simulink library "util_frame_rotation_lib"  (R2015b)
settings: Solver=ode45  SolverMode=SingleTasking  StartTime=0.0  StopTime=10.0  RelTol=1e-3
values from neighbouring files (symbols this model uses):
  D = P*P*P + Q*Q    [mci2lla.m]
undefined symbols (not defined in the file or in its folder): central_body_omega_dot, de_cos_coeff, de_t_poly, e10coeff, e11coeff, e12coeff, e13coeff, e1coeff, e2coeff, e3coeff, e4coeff, e5coeff, e6coeff, e7coeff, e8coeff, e9coeff, earth_moon_rotation_matrix_select, ini_epoch_seconds, ini_hour, ini_minute, ini_moon_rotation_rate, ini_quat_mcmf_to_topo, ini_seconds, ini_tgt_landing_mcmf_pos, omega_moon_iau_coeff, omega_pa_mat_init, ra_sin_coeff, ra_t_poly
undefined symbols (not defined in the file): central_body_flattening, central_body_radius, central_body_rotation_rate
libraries: util_quat_lib x42, util_info_lib x21, util_common_lib x18, util_frame_rotation_lib x14, simulink_extras x9, util_extra_lib x4, simulink x2, util_orbit_dynamics_lib x1
(part 1 of 2)
settings Model: Creator=Administrator  LastModifiedBy=Mark Agbayani
settings DataIOCC: SaveFormat=Array  SignalLoggingSaveFormat=ModelDataLogs
settings OptimizationCC: BlockReduction=off  BooleanDataType=off  ExpressionDepthLimit=2147483647
settings DebuggingCC: SaveWithParameterizedLinksMsg=none  UnderspecifiedInitializationDetection=Classic  MergeDetectMultiDrivingBlocksExec=none  SignalResolutionControl=TryResolveAllWithWarning  FcnCallInpInsideContextMsg=EnableAllAsWarning  StateNameClashWarn=warning  StrictBusMsg=Warning
settings HardwareCC: ProdBitPerPointer=32  ProdLargestAtomicFloat=None  ProdIntDivRoundTo=Undefined  ProdEndianess=Unspecified  ProdWordSize=32  ProdHWDeviceType=32-bit Generic  TargetUnknown=on
settings GRTTargetCC: GeneratePreprocessorConditionals=Disable all
settings ConfigComp: CovModelRefEnable=Off  CovSFcnEnable=off

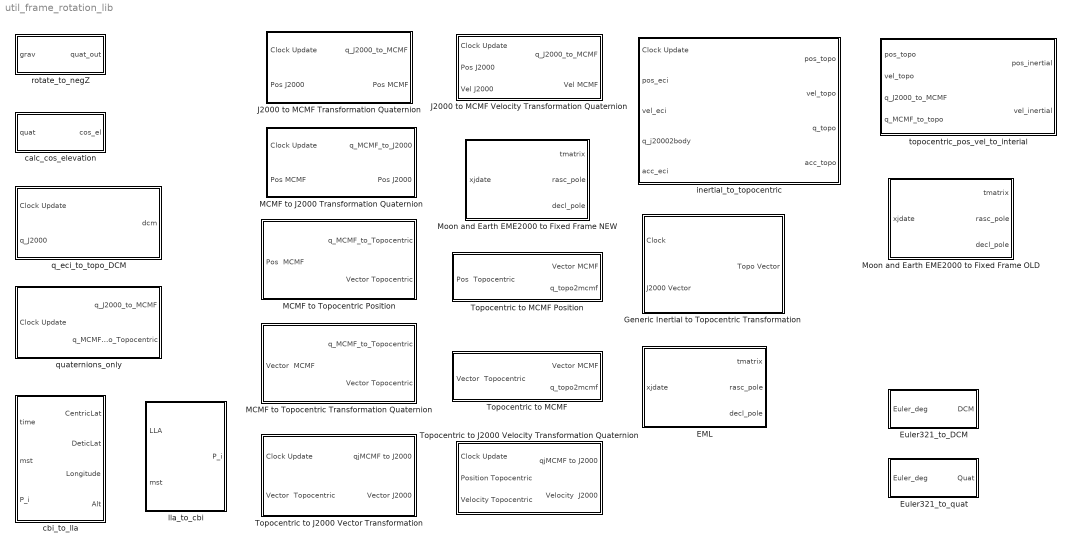
== system util_frame_rotation_lib ==
  EML : Subsystem
      mask Display:
      | color('blue')
      | text(0.05,0.02,'MoonEx',...
      |  	'HorizontalAlignment','Left',...
      | 	'VerticalAlignment','bottom')
  Euler321_to_DCM : Subsystem
  Euler321_to_quat : Subsystem
  Generic Inertial to Topocentric Transformation : Subsystem
  J2000 to MCMF Transformation Quaternion : Subsystem
      mask Display:
      | color('blue')
      | text(0.05,0.02,'MoonEx',...
      |  	'HorizontalAlignment','Left',...
      | 	'VerticalAlignment','bottom')
  J2000 to MCMF Velocity Transformation Quaternion : Subsystem
      mask Display:
      | color('blue')
      | text(0.05,0.02,'MoonEx',...
      |  	'HorizontalAlignment','Left',...
      | 	'VerticalAlignment','bottom')
  MCMF to J2000 Transformation Quaternion : Subsystem
  MCMF to Topocentric Position : Subsystem
      mask Display:
      | color('blue')
      | text(0.05,0.02,'MoonEx',...
      |  	'HorizontalAlignment','Left',...
      | 	'VerticalAlignment','bottom')
  MCMF to Topocentric Transformation Quaternion : Subsystem
      mask Display:
      | color('blue')
      | text(0.05,0.02,'MoonEx',...
      |  	'HorizontalAlignment','Left',...
      | 	'VerticalAlignment','bottom')
  Moon and Earth EME2000 to Fixed Frame NEW : Subsystem
      mask Display:
      | color('blue')
      | text(0.05,0.02,'MoonEx',...
      |  	'HorizontalAlignment','Left',...
      | 	'VerticalAlignment','bottom')
  Moon and Earth EME2000 to Fixed Frame OLD : Subsystem
      mask Display:
      | color('blue')
      | text(0.05,0.02,'MoonEx',...
      |  	'HorizontalAlignment','Left',...
      | 	'VerticalAlignment','bottom')
  "Topocentric to J2000 Vector Transformation " : Subsystem
      mask Display:
      | color('blue')
      | text(0.05,0.02,'MoonEx',...
      |  	'HorizontalAlignment','Left',...
      | 	'VerticalAlignment','bottom')
  Topocentric to J2000 Velocity Transformation Quaternion : Subsystem  TreatAsAtomicUnit=on
      mask Display:
      | color('blue')
      | text(0.05,0.02,'MoonEx',...
      |  	'HorizontalAlignment','Left',...
      | 	'VerticalAlignment','bottom')
  Topocentric to MCMF : Subsystem
      mask Display:
      | color('blue')
      | text(0.05,0.02,'MoonEx',...
      |  	'HorizontalAlignment','Left',...
      | 	'VerticalAlignment','bottom')
  Topocentric to MCMF Position : Subsystem
      mask Display:
      | color('blue')
      | text(0.05,0.02,'MoonEx',...
      |  	'HorizontalAlignment','Left',...
      | 	'VerticalAlignment','bottom')
  calc_cos_elevation : Subsystem
  cbi_to_lla : Subsystem  mask{a=central_body_radius, b=central_body_radius*(1-central_body_flattening), omega=central_body_rotation_rate(3)}
      mask prompts: a "Central Body Semi-major Axis (Equatorial Radius), a [m]"; b "Central Body Semi-minor Axis (Polar Radius), b [m]"; omega "Central Body Rotation Rate, omega [rad/s]"
      mask help:
      | FUNCTION cbi_to_lla
      |   Compute Detic Latitude, Centric Latitude, Longitude, and Detic Altitude
      |   from Central Body Inertial Coordinates
      |
      |   [latD, latC, lon, alt] = cbi_to_lla( P_i, t, mst)
      |
      | INPUTS
      |   P_i      [1x3]   [m]         Position in Central Body Inertial Frame
      |   mst      [1x1]   [degrees]   Mean Sidereal Time of Epoch
      |   time     [1x1]   [sec]       Time Since Epoch
      |
      | OUTPUTS
      |   latC     [1x1]   [deg]       Centric Latitude
      |   latD     [1x1]   [deg]       Detic Latitude
      |   lon      [1x1]   [deg]       Longitude
      |   alt      [1x1]   [m]         Detic Altitude
      mask init:
      | flatten = 1 - b/a;
      mask Display:
      | color('blue')
      | text(0.05,0.02,'MoonEx',...
      |  	'HorizontalAlignment','Left',...
      | 	'VerticalAlignment','bottom')
  inertial_to_topocentric : Subsystem
      mask Display:
      | color('blue')
      | text(0.05,0.02,'MoonEx',...
      |  	'HorizontalAlignment','Left',...
      | 	'VerticalAlignment','bottom')
  lla_to_cbi : Subsystem  mask{a=central_body_radius, b=central_body_radius*(1-central_body_flattening)}
      mask prompts: a "Central Body Semi-major Axis (Equatorial Radius), a [m]"; b "Central Body Semi-minor Axis (Polar Radius), b [m]"
      mask help:
      | FUNCTION lla_to_cbi
      |   Converts Detic Latitude, Longitude, and Altitude
      |   to Central Body Inertial Coordinates.
      |
      |   P_i = lla_to_cbi( LLA, mst)
      |
      | INPUTS
      |   LLA      [1x3]   [deg deg m]    Detic Lattitude, Longitude, Altitude
      |   mst      [1x1]   [degrees]      Mean Sidereal Time of Epoch
      |
      | OUTPUTS
      |   P_i      [1x3]   [m]            Position in Central Body Inertial Frame
      mask init:
      | flatten = 1 - b/a;
      mask Display:
      | color('blue')
      | text(0.05,0.02,'MoonEx',...
      |  	'HorizontalAlignment','Left',...
      | 	'VerticalAlignment','bottom')
  q_eci_to_topo_DCM : Subsystem
      mask Display:
      | color('blue')
      | text(0.05,0.02,'MoonEx',...
      |  	'HorizontalAlignment','Left',...
      | 	'VerticalAlignment','bottom')
  quaternions_only : Subsystem
      mask Display:
      | color('blue')
      | text(0.05,0.02,'MoonEx',...
      |  	'HorizontalAlignment','Left',...
      | 	'VerticalAlignment','bottom')
  rotate_to_negZ : Subsystem
  topocentric_pos_vel_to_interial : Subsystem
      mask Display:
      | color('blue')
      | text(0.05,0.02,'MoonEx',...
      |  	'HorizontalAlignment','Left',...
      | 	'VerticalAlignment','bottom')

== system util_frame_rotation_lib/EML ==
  xjdate : Inport
  EME2000 (J2000) to Moon Centered Moon Fixed (MCMF) : MATLAB Function  TreatAsAtomicUnit=on
  Library Information : util_info_lib/Library Information  owner='NONE'
  Moon Rotation Rate vector : Constant  Value=ini_moon_rotation_rate
  tmatrix : Outport
  rasc_pole : Outport  Port=2
  decl_pole : Outport  Port=3
  wires:
  EME2000 (J2000) to Moon Centered Moon Fixed (MCMF)/1(tmatrix) -> tmatrix/1
  EME2000 (J2000) to Moon Centered Moon Fixed (MCMF)/2(rasc_pole) -> rasc_pole/1
  EME2000 (J2000) to Moon Centered Moon Fixed (MCMF)/3(decl_pole) -> decl_pole/1
  xjdate/1 -> EME2000 (J2000) to Moon Centered Moon Fixed (MCMF)/1(xjdate)
  Moon Rotation Rate vector/1 -> EME2000 (J2000) to Moon Centered Moon Fixed (MCMF)/2(moonrotationrate)

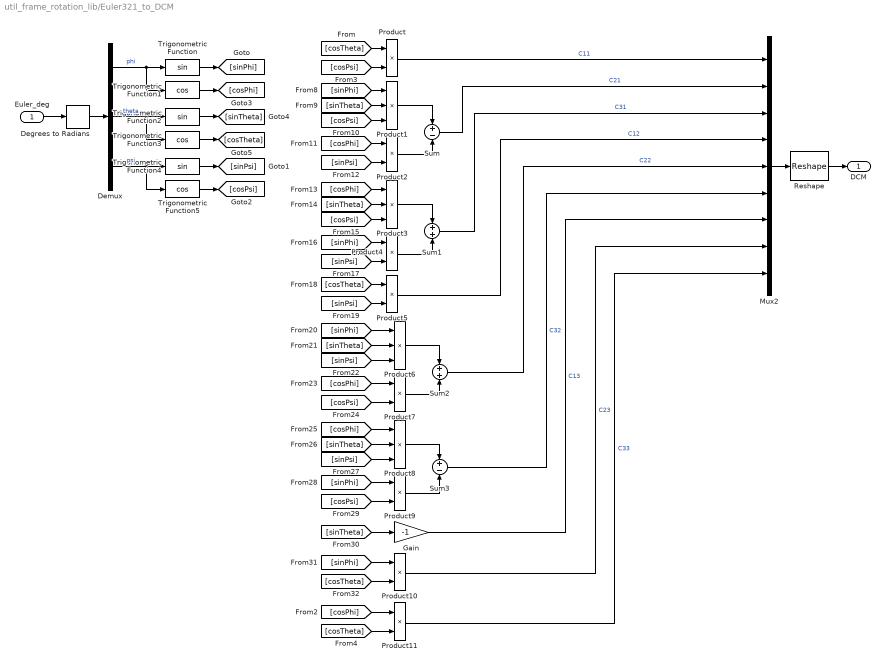
== system util_frame_rotation_lib/Euler321_to_DCM ==
  Euler_deg : Inport
  Degrees to Radians : simulink_extras/Transformations/Degrees to Radians
  Demux : Demux  Outputs=3
  Gain : Gain  Gain=-1
  Mux2 : Mux  Inputs=9
  Product{,2,4..5,7,9..11} (8 alike) : Product  RndMeth=Zero
  Product{1,3,6,8} (4 alike) : Product  Inputs=3  RndMeth=Zero
  Reshape : Reshape  OutputDimensionality=Customize  OutputDimensions=[3,3]
  Sum : Sum  Inputs=+|-
  Sum1 : Sum  Inputs=+|+
  Sum2 : Sum  Inputs=+|+
  Sum3 : Sum  Inputs=+|-
  Trigonometric Function : Trigonometry
  Trigonometric Function1 : Trigonometry  Operator=cos
  Trigonometric Function2 : Trigonometry
  Trigonometric Function3 : Trigonometry  Operator=cos
  Trigonometric Function4 : Trigonometry
  Trigonometric Function5 : Trigonometry  Operator=cos
  DCM : Outport
  wires:
  Degrees to Radians/1 -> Demux/1
  Demux/1 -> Trigonometric Function/1, Trigonometric Function1/1  "phi"
  Demux/2 -> Trigonometric Function3/1, Trigonometric Function2/1  "theta"
  Demux/3 -> Trigonometric Function4/1, Trigonometric Function5/1  "psi"
  Trigonometric Function/1 -> [sinPhi]
  Trigonometric Function1/1 -> [cosPhi]
  Trigonometric Function2/1 -> [sinTheta]
  Trigonometric Function3/1 -> [cosTheta]
  Trigonometric Function4/1 -> [sinPsi]
  Trigonometric Function5/1 -> [cosPsi]
  [cosTheta] -> Product/1
  [cosPsi] -> Product/2
  Product/1 -> Mux2/1  "C11"
  Product1/1 -> Sum/1
  Product2/1 -> Sum/2
  [sinPhi] -> Product1/1
  [sinTheta] -> Product1/2
  [cosPsi] -> Product1/3
  [cosPhi] -> Product2/1
  [sinPsi] -> Product2/2
  Sum/1 -> Mux2/2  "C21"
  Product3/1 -> Sum1/1
  Product4/1 -> Sum1/2
  Sum1/1 -> Mux2/3  "C31"
  [cosPhi] -> Product3/1
  [sinTheta] -> Product3/2
  [cosPsi] -> Product3/3
  [sinPhi] -> Product4/1
  [sinPsi] -> Product4/2
  [cosTheta] -> Product5/1
  [sinPsi] -> Product5/2
  Product5/1 -> Mux2/4  "C12"
  Product6/1 -> Sum2/1
  Product7/1 -> Sum2/2
  [sinPhi] -> Product6/1
  [sinTheta] -> Product6/2
  [sinPsi] -> Product6/3
  [cosPhi] -> Product7/1
  [cosPsi] -> Product7/2
  Sum2/1 -> Mux2/5  "C22"
  Product8/1 -> Sum3/1
  Product9/1 -> Sum3/2
  [cosPhi] -> Product8/1
  [sinTheta] -> Product8/2
  [sinPsi] -> Product8/3
  [sinPhi] -> Product9/1
  [cosPsi] -> Product9/2
  Sum3/1 -> Mux2/6  "C32"
  Gain/1 -> Mux2/7  "C13"
  [sinTheta] -> Gain/1
  [sinPhi] -> Product10/1
  [cosTheta] -> Product10/2
  Product10/1 -> Mux2/8  "C23"
  [cosPhi] -> Product11/1
  [cosTheta] -> Product11/2
  Product11/1 -> Mux2/9  "C33"
  Euler_deg/1 -> Degrees to Radians/1
  Mux2/1 -> Reshape/1
  Reshape/1 -> DCM/1

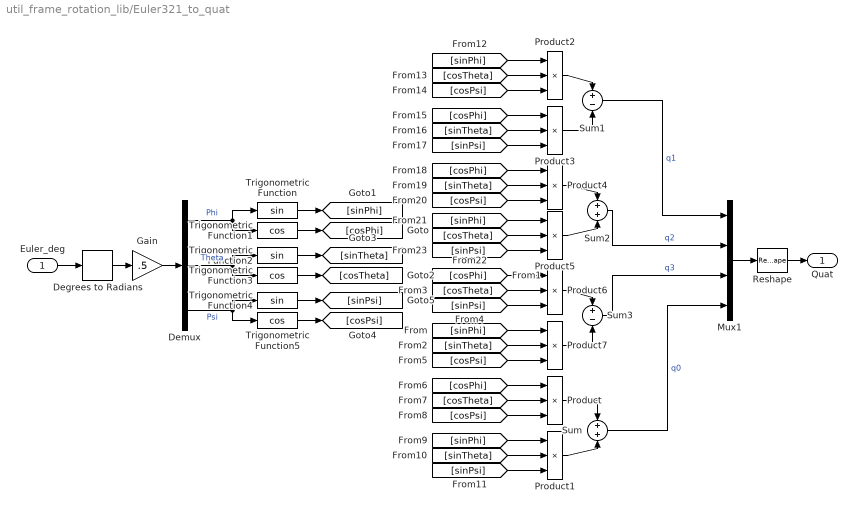
== system util_frame_rotation_lib/Euler321_to_quat ==
  Euler_deg : Inport
  Degrees to Radians : simulink_extras/Transformations/Degrees to Radians
  Demux : Demux  Outputs=3
  Gain : Gain  Gain=.5
  Mux1 : Mux
  Product{,1..7} (8 alike) : Product  Inputs=3  RndMeth=Zero
  Reshape : Reshape
  Sum : Sum  Inputs=+|+
  Sum1 : Sum  Inputs=+|-
  Sum2 : Sum  Inputs=+|+
  Sum3 : Sum  Inputs=+|-
  Trigonometric Function : Trigonometry
  Trigonometric Function1 : Trigonometry  Operator=cos
  Trigonometric Function2 : Trigonometry
  Trigonometric Function3 : Trigonometry  Operator=cos
  Trigonometric Function4 : Trigonometry
  Trigonometric Function5 : Trigonometry  Operator=cos
  Quat : Outport
  wires:
  Reshape/1 -> Quat/1
  Mux1/1 -> Reshape/1
  Euler_deg/1 -> Degrees to Radians/1
  [cosPsi] -> Product7/3
  [sinTheta] -> Product7/2
  [sinPhi] -> Product7/1
  [sinPsi] -> Product6/3
  [cosTheta] -> Product6/2
  [cosPhi] -> Product6/1
  Product6/1 -> Sum3/1
  Product7/1 -> Sum3/2
  Product5/1 -> Sum2/2
  [sinPsi] -> Product5/3
  [cosTheta] -> Product5/2
  [sinPhi] -> Product5/1
  Product4/1 -> Sum2/1
  [cosPsi] -> Product4/3
  [sinTheta] -> Product4/2
  [cosPhi] -> Product4/1
  Product3/1 -> Sum1/2
  [sinPsi] -> Product3/3
  [sinTheta] -> Product3/2
  [cosPhi] -> Product3/1
  Product2/1 -> Sum1/1
  [cosPsi] -> Product2/3
  [cosTheta] -> Product2/2
  [sinPhi] -> Product2/1
  [sinPsi] -> Product1/3
  [sinTheta] -> Product1/2
  [sinPhi] -> Product1/1
  Product1/1 -> Sum/2
  Product/1 -> Sum/1
  [cosPsi] -> Product/3
  [cosTheta] -> Product/2
  [cosPhi] -> Product/1
  Trigonometric Function5/1 -> [cosPsi]
  Trigonometric Function4/1 -> [sinPsi]
  Trigonometric Function3/1 -> [cosTheta]
  Trigonometric Function2/1 -> [sinTheta]
  Trigonometric Function1/1 -> [cosPhi]
  Trigonometric Function/1 -> [sinPhi]
  Demux/3 -> Trigonometric Function5/1, Trigonometric Function4/1  "Psi"
  Demux/2 -> Trigonometric Function3/1, Trigonometric Function2/1  "Theta"
  Demux/1 -> Trigonometric Function1/1, Trigonometric Function/1  "Phi"
  Gain/1 -> Demux/1
  Sum1/1 -> Mux1/1  "q1"
  Sum2/1 -> Mux1/2  "q2"
  Sum3/1 -> Mux1/3  "q3"
  Sum/1 -> Mux1/4  "q0"
  Degrees to Radians/1 -> Gain/1

== system util_frame_rotation_lib/Generic Inertial to Topocentric Transformation ==
  Clock : Inport
  J2000 Vector : Inport  Port=2
  J2000 to MCMF Transformation Quaternion1 : util_frame_rotation_lib/J2000 to MCMF  Transformation Quaternion  SystemSampleTime=-1
  Library Information : util_info_lib/Library Information  owner='NONE'
  MCMF to Topocentric Transformation Quaternion : util_frame_rotation_lib/MCMF to Topocentric  Transformation Quaternion  SystemSampleTime=-1
  Terminator : Terminator
  Terminator1 : Terminator
  Topo Vector : Outport
  wires:
  J2000 to MCMF Transformation Quaternion1/2 -> MCMF to Topocentric Transformation Quaternion/1
  J2000 to MCMF Transformation Quaternion1/1 -> Terminator/1
  J2000 Vector/1 -> J2000 to MCMF Transformation Quaternion1/2
  MCMF to Topocentric Transformation Quaternion/2 -> Topo Vector/1
  Clock/1 -> J2000 to MCMF Transformation Quaternion1/1
  MCMF to Topocentric Transformation Quaternion/1 -> Terminator1/1

== system util_frame_rotation_lib/J2000 to MCMF Transformation Quaternion ==
  Clock Update : Inport
  Pos J2000 : Inport  Port=2
  Add : Sum
  Divide : Product  Inputs=*/
  Library Information : util_info_lib/Library Information  owner='NONE'
  Moon and Earth EME2000 to Fixed Frame NEW : util_frame_rotation_lib/Moon and Earth  EME2000 to Fixed Frame NEW  SystemSampleTime=-1
  "Number of Days From Start of Julian Date to Jan 1, 2000 12:00:00" : Constant  Value=2451545
  Number of Seconds Per Day : Constant  Description=|  Value=86400
      | Number of Seconds                   
      | July 4, 2014 22:40:00 UTC           
      | Calculate on Web Site:              
      | www.mbari.org/staff/rich/utccalc.htm
  Terminator1 : Terminator
  Terminator5 : Terminator
  quaternion_frame_transformation : util_quat_lib/quaternion_frame_transformation  SystemSampleTime=-1
  rotm_to_quaternion EME2000 to MCMF : util_extra_lib/rotm_to_quaternion
  q_J2000_to_MCMF : Outport
  Pos MCMF : Outport  Port=2
  wires:
  Moon and Earth EME2000 to Fixed Frame NEW/1 -> rotm_to_quaternion EME2000 to MCMF/1
  Number of Seconds Per Day/1 -> Divide/2
  rotm_to_quaternion EME2000 to MCMF/1 -> quaternion_frame_transformation/2, q_J2000_to_MCMF/1
  Clock Update/1 -> Divide/1  "Seconds Since Jan 1, 2000  12:00:00"
  quaternion_frame_transformation/1 -> Pos MCMF/1
  "Number of Days From Start of Julian Date to Jan 1, 2000 12:00:00"/1 -> Add/2
  Moon and Earth EME2000 to Fixed Frame NEW/2 -> Terminator5/1
  Moon and Earth EME2000 to Fixed Frame NEW/3 -> Terminator1/1
  Add/1 -> Moon and Earth EME2000 to Fixed Frame NEW/1
  Divide/1 -> Add/1
  Pos J2000/1 -> quaternion_frame_transformation/1

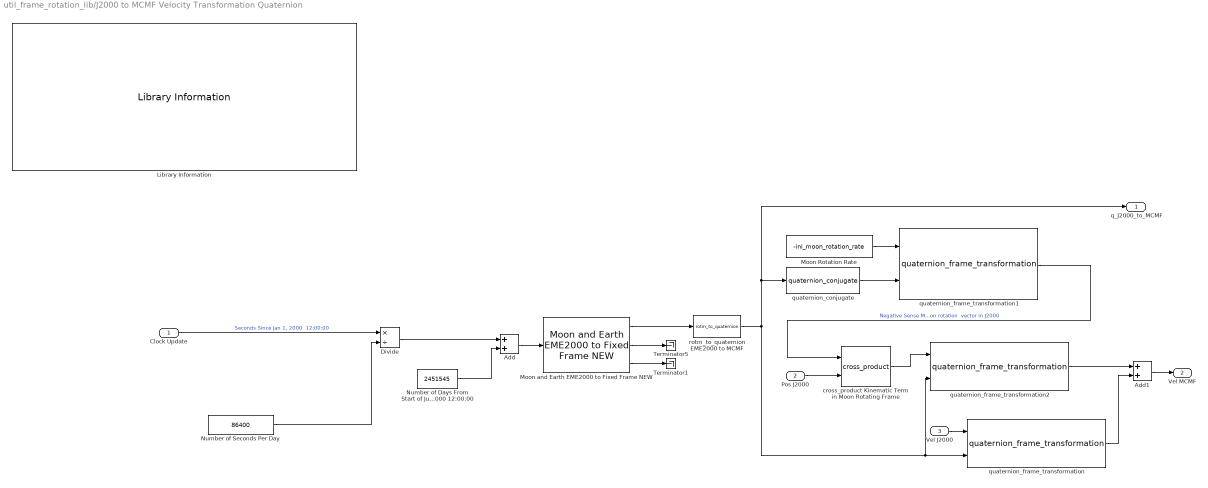
== system util_frame_rotation_lib/J2000 to MCMF Velocity Transformation Quaternion ==
  Clock Update : Inport
  Pos J2000 : Inport  Port=2
  Vel J2000 : Inport  Port=3
  Add : Sum
  Add1 : Sum
  Divide : Product  Inputs=*/
  Library Information : util_info_lib/Library Information  owner='NONE'
  Moon Rotation Rate : Constant  Value=-ini_moon_rotation_rate
  Moon and Earth EME2000 to Fixed Frame NEW : util_frame_rotation_lib/Moon and Earth  EME2000 to Fixed Frame NEW  SystemSampleTime=-1
  "Number of Days From Start of Julian Date to Jan 1, 2000 12:00:00" : Constant  Value=2451545
  Number of Seconds Per Day : Constant  Description=|  Value=86400
      | Number of Seconds                   
      | July 4, 2014 22:40:00 UTC           
      | Calculate on Web Site:              
      | www.mbari.org/staff/rich/utccalc.htm
  Terminator1 : Terminator
  Terminator5 : Terminator
  cross_product Kinematic Term in Moon Rotating Frame : util_common_lib/cross_product  SystemSampleTime=-1
  quaternion_conjugate : util_quat_lib/quaternion_conjugate  SystemSampleTime=-1
  quaternion_frame_transformation : util_quat_lib/quaternion_frame_transformation  SystemSampleTime=-1
  quaternion_frame_transformation1 : util_quat_lib/quaternion_frame_transformation  SystemSampleTime=-1
  quaternion_frame_transformation2 : util_quat_lib/quaternion_frame_transformation  SystemSampleTime=-1
  rotm_to_quaternion EME2000 to MCMF : util_extra_lib/rotm_to_quaternion
  q_J2000_to_MCMF : Outport
  Vel MCMF : Outport  Port=2
  wires:
  Vel J2000/1 -> quaternion_frame_transformation/1
  Divide/1 -> Add/1
  Add/1 -> Moon and Earth EME2000 to Fixed Frame NEW/1
  Moon and Earth EME2000 to Fixed Frame NEW/3 -> Terminator1/1
  Moon and Earth EME2000 to Fixed Frame NEW/2 -> Terminator5/1
  "Number of Days From Start of Julian Date to Jan 1, 2000 12:00:00"/1 -> Add/2
  Clock Update/1 -> Divide/1  "Seconds Since Jan 1, 2000  12:00:00"
  rotm_to_quaternion EME2000 to MCMF/1 -> quaternion_frame_transformation2/2, quaternion_frame_transformation/2, q_J2000_to_MCMF/1, quaternion_conjugate/1
  Number of Seconds Per Day/1 -> Divide/2
  Moon and Earth EME2000 to Fixed Frame NEW/1 -> rotm_to_quaternion EME2000 to MCMF/1
  Moon Rotation Rate/1 -> quaternion_frame_transformation1/1
  quaternion_conjugate/1 -> quaternion_frame_transformation1/2
  quaternion_frame_transformation1/1 -> cross_product Kinematic Term in Moon Rotating Frame/1  "Negative Sense Moon rotation  vector in J2000"
  Add1/1 -> Vel MCMF/1
  quaternion_frame_transformation/1 -> Add1/2
  Pos J2000/1 -> cross_product Kinematic Term in Moon Rotating Frame/2
  quaternion_frame_transformation2/1 -> Add1/1
  cross_product Kinematic Term in Moon Rotating Frame/1 -> quaternion_frame_transformation2/1

== system util_frame_rotation_lib/MCMF to J2000 Transformation Quaternion ==
  note: Calculate on Web Site:
      | www.mbari.org/staff/rich/utccalc.htm
  Clock Update : Inport
  Pos MCMF : Inport  Port=2
  Add : Sum
  Divide : Product  Inputs=*/
  Library Information : util_info_lib/Library Information  owner='NONE'
  Moon and Earth EME2000 to Fixed Frame NEW : util_frame_rotation_lib/Moon and Earth  EME2000 to Fixed Frame NEW  SystemSampleTime=-1
  "Number of Days From Start of Julian Date to Jan 1, 2000 12:00:00" : Constant  Value=2451545
  Number of Seconds Per Day : Constant  Description=|  Value=86400
      | Number of Seconds                   
      | July 4, 2014 22:40:00 UTC           
      | Calculate on Web Site:              
      | www.mbari.org/staff/rich/utccalc.htm
  Terminator1 : Terminator
  Terminator5 : Terminator
  quaternion_conjugate : util_quat_lib/quaternion_conjugate  SystemSampleTime=-1
  quaternion_frame_transformation : util_quat_lib/quaternion_frame_transformation  SystemSampleTime=-1
  rotm_to_quaternion EME2000 to MCMF : util_extra_lib/rotm_to_quaternion
  q_MCMF_to_J2000 : Outport
  Pos J2000 : Outport  Port=2
  wires:
  Pos MCMF/1 -> quaternion_frame_transformation/1
  Divide/1 -> Add/1
  Add/1 -> Moon and Earth EME2000 to Fixed Frame NEW/1
  Moon and Earth EME2000 to Fixed Frame NEW/3 -> Terminator1/1
  Moon and Earth EME2000 to Fixed Frame NEW/2 -> Terminator5/1
  "Number of Days From Start of Julian Date to Jan 1, 2000 12:00:00"/1 -> Add/2
  quaternion_frame_transformation/1 -> Pos J2000/1
  Clock Update/1 -> Divide/1  "Seconds Since Jan 1, 2000  12:00:00"
  rotm_to_quaternion EME2000 to MCMF/1 -> quaternion_conjugate/1
  Number of Seconds Per Day/1 -> Divide/2
  Moon and Earth EME2000 to Fixed Frame NEW/1 -> rotm_to_quaternion EME2000 to MCMF/1
  quaternion_conjugate/1 -> quaternion_frame_transformation/2, q_MCMF_to_J2000/1

== system util_frame_rotation_lib/MCMF to Topocentric Position ==
  Pos  MCMF : Inport
  Constant10 : Constant  Value=ini_tgt_landing_mcmf_pos
  Library Information : util_info_lib/Library Information  owner='NONE'
  Moon Rotation Rate in MCMF : Constant  Value=ini_quat_mcmf_to_topo
  Subtract1 : Sum  Inputs=-+
  quaternion_frame_transformation1 : util_quat_lib/quaternion_frame_transformation  SystemSampleTime=-1
  q_MCMF_to_Topocentric : Outport
  Vector Topocentric : Outport  Port=2
  wires:
  Moon Rotation Rate in MCMF/1 -> quaternion_frame_transformation1/2, q_MCMF_to_Topocentric/1
  quaternion_frame_transformation1/1 -> Vector Topocentric/1
  Constant10/1 -> Subtract1/1
  Pos  MCMF/1 -> Subtract1/2
  Subtract1/1 -> quaternion_frame_transformation1/1

== system util_frame_rotation_lib/MCMF to Topocentric Transformation Quaternion ==
  Vector  MCMF : Inport
  Library Information : util_info_lib/Library Information  owner='NONE'
  Moon Rotation Rate in MCMF : Constant  Value=ini_quat_mcmf_to_topo
  quaternion_frame_transformation1 : util_quat_lib/quaternion_frame_transformation  SystemSampleTime=-1
  q_MCMF_to_Topocentric : Outport
  Vector Topocentric : Outport  Port=2
  wires:
  Moon Rotation Rate in MCMF/1 -> quaternion_frame_transformation1/2, q_MCMF_to_Topocentric/1
  quaternion_frame_transformation1/1 -> Vector Topocentric/1
  Vector  MCMF/1 -> quaternion_frame_transformation1/1

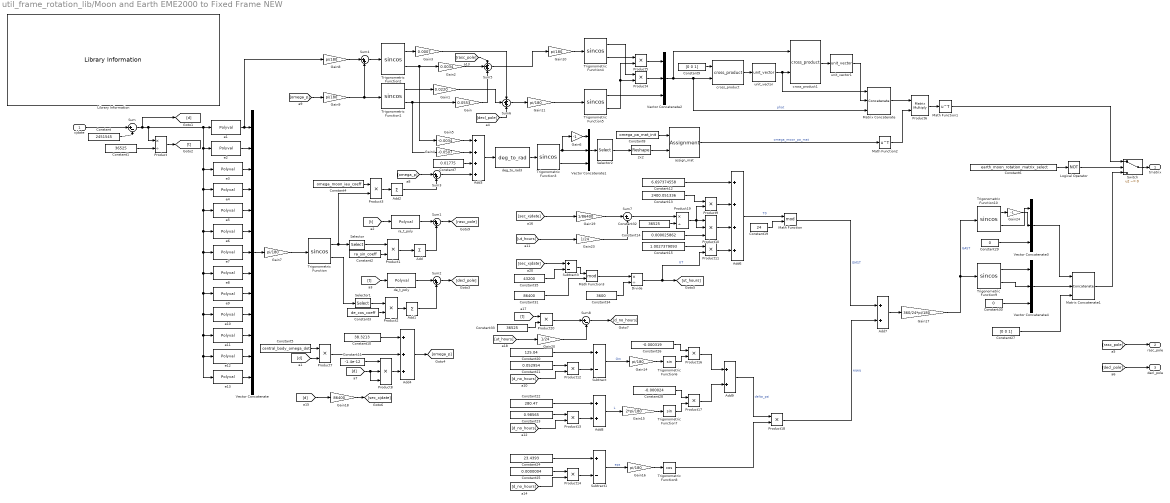
== system util_frame_rotation_lib/Moon and Earth EME2000 to Fixed Frame NEW ==
  xjdate : Inport
  2x2 : Reshape  OutputDimensionality=Customize  OutputDimensions=[2,2]
  Add : Sum  Inputs=+
  Add1 : Sum  Inputs=+
  Add2 : Sum  Inputs=+
  Add3 : Sum  Inputs=4
  Add4 : Sum  Inputs=3
  Add6 : Sum  Inputs=4
  Add7 : Sum  Inputs=2
  Add8 : Sum  Inputs=2
  Add9 : Sum  Inputs=2
  Constant : Constant  Value=2451545
  Constant1 : Constant  Value=36525
  Constant10 : Constant  Value=38.3213
  Constant11 : Constant  Value=-1.4e-12
  Constant12 : Constant  Value=6.697374558
  Constant13 : Constant  Value=2400.051336
  Constant14 : Constant  Value=0.000025862
  Constant15 : Constant  Value=1.0027379093
  Constant19 : Constant  Value=24
  Constant2 : Constant  Value=ra_sin_coeff
  Constant20 : Constant  Value=125.04
  Constant21 : Constant  Value=0.052954
  Constant22 : Constant  Value=280.47
  Constant23 : Constant  Value=0.98565
  Constant24 : Constant  Value=23.4393
  Constant25 : Constant  Value=0.0000004
  Constant26 : Constant  Value=-0.000319
  Constant27 : Constant  Value=[0 0 1]
  Constant28 : Constant  Value=-0.000024
  Constant29 : Constant  Value=0
  Constant3 : Constant  Value=de_cos_coeff
  Constant30 : Constant  Value=0
  Constant31 : Constant  Value=86400
  Constant32 : Constant  Value=36525
  Constant33 : Constant  Value=36525
  Constant34 : Constant  Value=3600
  Constant35 : Constant  Value=43200
  Constant4 : Constant  Value=omega_moon_iau_coeff
  Constant5 : Constant  Value=central_body_omega_dot
  Constant6 : Constant  Value=earth_moon_rotation_matrix_select
  Constant7 : Constant  Value=0.01775
  Constant8 : Constant  Value=omega_pa_mat_init
  Constant9 : Constant  Value=[0 0 1]
  Divide : Product  Inputs=*/
  Gain : Gain  Gain=0.0553
  Gain1 : Gain  Gain=0.0220
  Gain{7..11,14,16} (7 alike) : Gain  Gain=pi/180
  Gain15 : Gain  Gain=2*pi/180
  Gain17 : Gain  Gain=360/24*pi/180
  Gain18 : Gain  Gain=86400
  Gain19 : Gain  Gain=1/86400
  Gain2 : Gain  Gain=0.0034
  Gain20 : Gain  Gain=1/24
  Gain23 : Gain  Gain=1/24
  Gain24 : Gain  Gain=-1
  Gain3 : Gain  Gain=0.0007
  Gain4 : Gain  Gain=-0.0507
  Gain5 : Gain  Gain=-0.0034
  Gain6 : Gain  Gain=-1
  Library Information : util_info_lib/Library Information  owner='escrane'
  Logical Operator : Logic  Operator=NOT  AllPortsSameDT=off  OutDataTypeStr=boolean
  Math Function : Math  Operator=mod  SaturateOnIntegerOverflow=on
  Math Function1 : Math  Operator=transpose  SaturateOnIntegerOverflow=on
  Math Function2 : Math  Operator=transpose  SaturateOnIntegerOverflow=on
  Math Function3 : Math  Operator=mod  SaturateOnIntegerOverflow=on
  Matrix Concatenate : Concatenate  NumInputs=3  Mode=Multidimensional array  ConcatenateDimension=2
  Matrix Concatenate1 : Concatenate  NumInputs=3  Mode=Multidimensional array  ConcatenateDimension=2
  Product : Product  Inputs=*/
  Product{1..5,7,9,11..14,16..18,20} (15 alike) : Product
  Product10 : Product  Inputs=3
  Product19 : Product  Inputs=*/
  Product6 : Product  Multiplication=Matrix(*)
  Product8 : Product  Inputs=3
  Selector : Selector  InputPortWidth=13  IndexOptions=Index vector (dialog)  Indices=[1 2 3 4 6 10 13]  OutputSizes=1
  Selector1 : Selector  InputPortWidth=13  IndexOptions=Index vector (dialog)  Indices=[1 2 3 4 6 7 10 13]  OutputSizes=1
  Selector2 : Selector  InputPortWidth=3  IndexOptions=Index vector (dialog)  Indices=[3 1 2 3]  OutputSizes=1
  Subtract : Sum  Inputs=+-
  Subtract1 : Sum  Inputs=+-
  Subtract3 : Sum  Inputs=+-
  Sum : Sum  Inputs=|+-
  Sum{1..4} (4 alike) : Sum  Inputs=|++
  Sum5 : Sum  Inputs=+++
  Sum6 : Sum  Inputs=+++
  Sum7 : Sum  Inputs=|+-
  Sum8 : Sum  Inputs=|+-
  Switch : Switch  Criteria=u2 ~= 0
  Trigonometric Function{,1..5,9..10} (8 alike) : Trigonometry  Operator=sincos
  Trigonometric Function6 : Trigonometry
  Trigonometric Function7 : Trigonometry
  Trigonometric Function8 : Trigonometry  Operator=cos
  Vector Concatenate : Concatenate  NumInputs=13
  Vector Concatenate{1..4} (4 alike) : Concatenate  NumInputs=3
  assign_mat : Assignment  NumberOfDimensions=2  IndexOptions=Index vector (dialog),Index vector (dialog)  Indices=[1 2],[1 2]  OutputSizes=1,1
  cross_product : util_common_lib/cross_product  SystemSampleTime=-1
  cross_product1 : util_common_lib/cross_product  SystemSampleTime=-1
  de_t_poly : Polyval  Coefs=de_t_poly
  deg_to_rad3 : util_common_lib/deg_to_rad  SystemSampleTime=-1
  e1 : Polyval  Coefs=e1coeff
  e10 : Polyval  Coefs=e10coeff
  e11 : Polyval  Coefs=e11coeff
  e12 : Polyval  Coefs=e12coeff
  e13 : Polyval  Coefs=e13coeff
  e2 : Polyval  Coefs=e2coeff
  e3 : Polyval  Coefs=e3coeff
  e4 : Polyval  Coefs=e4coeff
  e5 : Polyval  Coefs=e5coeff
  e6 : Polyval  Coefs=e6coeff
  e7 : Polyval  Coefs=e7coeff
  e8 : Polyval  Coefs=e8coeff
  e9 : Polyval  Coefs=e9coeff
  ra_t_poly : Polyval  Coefs=ra_t_poly
  unit_vector : util_common_lib/unit_vector  SystemSampleTime=-1
  unit_vector1 : util_common_lib/unit_vector  SystemSampleTime=-1
  tmatrix : Outport
  rasc_pole : Outport  Port=2
  decl_pole : Outport  Port=3
  wires:
  [decl_pole] -> decl_pole/1
  [rasc_pole] -> rasc_pole/1
  Math Function2/1 -> Product6/2
  Trigonometric Function5/2 -> Product5/2, Product4/2
  Gain3/1 -> Sum6/1
  Gain1/1 -> Sum6/2
  Gain2/1 -> Sum5/2
  Gain/1 -> Sum5/3
  Product6/1 -> Math Function1/1
  Matrix Concatenate/1 -> Product6/1
  unit_vector1/1 -> Matrix Concatenate/2
  cross_product1/1 -> unit_vector1/1
  unit_vector/1 -> cross_product1/2, Matrix Concatenate/1
  cross_product/1 -> unit_vector/1
  Constant9/1 -> cross_product/1
  Vector Concatenate2/1 -> cross_product/2, Matrix Concatenate/3, cross_product1/1  "phat"
  Product4/1 -> Vector Concatenate2/2
  Product5/1 -> Vector Concatenate2/1
  Trigonometric Function4/2 -> Product5/1
  Trigonometric Function5/1 -> Vector Concatenate2/3
  Trigonometric Function4/1 -> Product4/1
  Gain11/1 -> Trigonometric Function5/1
  Gain10/1 -> Trigonometric Function4/1
  assign_mat/1 -> Math Function2/1  "omega_moon_pa_mat"
  Constant8/1 -> assign_mat/1
  2x2/1 -> assign_mat/2
  Selector2/1 -> 2x2/1
  Vector Concatenate1/1 -> Selector2/1
  Gain6/1 -> Vector Concatenate1/1
  Trigonometric Function3/1 -> Vector Concatenate1/2, Gain6/1
  Trigonometric Function3/2 -> Vector Concatenate1/3
  deg_to_rad3/1 -> Trigonometric Function3/1
  Add3/1 -> deg_to_rad3/1
  Constant7/1 -> Add3/3
  Gain4/1 -> Add3/2
  Gain5/1 -> Add3/1
  Sum6/1 -> Gain11/1
  Sum5/1 -> Gain10/1
  [rasc_pole] -> Sum5/1
  [decl_pole] -> Sum6/3
  Trigonometric Function2/2 -> Gain5/1, Gain2/1
  Trigonometric Function2/1 -> Gain3/1
  Trigonometric Function1/1 -> Gain1/1
  Trigonometric Function1/2 -> Gain/1, Gain4/1
  Sum4/1 -> Trigonometric Function2/1
  Gain8/1 -> Sum4/1
  Gain9/1 -> Trigonometric Function1/1, Sum4/2
  [omega_p] -> Gain9/1
  Sum3/1 -> Add3/4
  Add2/1 -> Sum3/2
  Product3/1 -> Add2/1
  Constant4/1 -> Product3/1
  Sum2/1 -> [decl_pole]
  Add1/1 -> Sum2/2
  de_t_poly/1 -> Sum2/1
  Product2/1 -> Add1/1
  Constant3/1 -> Product2/2
  Selector1/1 -> Product2/1
  [t] -> de_t_poly/1
  Sum1/1 -> [rasc_pole]
  Add/1 -> Sum1/2
  ra_t_poly/1 -> Sum1/1
  Product1/1 -> Add/1
  Constant2/1 -> Product1/2
  Selector/1 -> Product1/1
  [t] -> ra_t_poly/1
  Trigonometric Function/2 -> Selector1/1
  Trigonometric Function/1 -> Selector/1, Product3/2
  Gain7/1 -> Trigonometric Function/1
  Vector Concatenate/1 -> Gain7/1
  e13/1 -> Vector Concatenate/13
  e12/1 -> Vector Concatenate/12
  e11/1 -> Vector Concatenate/11
  e10/1 -> Vector Concatenate/10
  e9/1 -> Vector Concatenate/9
  e8/1 -> Vector Concatenate/8
  e7/1 -> Vector Concatenate/7
  e6/1 -> Vector Concatenate/6
  e5/1 -> Vector Concatenate/5
  e4/1 -> Vector Concatenate/4
  e3/1 -> Vector Concatenate/3
  e2/1 -> Vector Concatenate/2
  e1/1 -> Vector Concatenate/1, Gain8/1
  Sum/1 -> [d], Product/1, e1/1, e2/1, e3/1, e4/1, e5/1, e6/1, e7/1, e8/1, e9/1, e11/1, e12/1, e13/1, e10/1
  Product/1 -> [t]
  Constant1/1 -> Product/2
  Constant/1 -> Sum/2
  xjdate/1 -> Sum/1
  Constant5/1 -> Product7/1
  [d] -> Product7/2
  Constant11/1 -> Product8/1
  [d] -> Product8/3, Product8/2
  Constant10/1 -> Add4/1
  Product7/1 -> Add4/2
  Product8/1 -> Add4/3
  Add4/1 -> [omega_p]
  [omega_p] -> Sum3/1
  Constant6/1 -> Logical Operator/1
  Logical Operator/1 -> Switch/2
  Switch/1 -> tmatrix/1
  Math Function1/1 -> Switch/1
  Constant12/1 -> Add6/1
  Constant13/1 -> Product9/1
  Product9/1 -> Add6/2
  Constant14/1 -> Product10/3
  Product10/1 -> Add6/3
  Constant15/1 -> Product11/1
  Divide/1 -> Product11/2, [ut_hours]  "UT"
  Product11/1 -> Add6/4
  Constant19/1 -> Math Function/2
  Add6/1 -> Math Function/1  "T0"
  Constant20/1 -> Subtract/1
  Product12/1 -> Subtract/2
  Constant21/1 -> Product12/1
  Constant22/1 -> Add8/1
  Product13/1 -> Add8/2
  Constant23/1 -> Product13/1
  Constant24/1 -> Subtract1/1
  Product14/1 -> Subtract1/2
  Constant25/1 -> Product14/1
  [d_no_hours] -> Product14/2
  Subtract/1 -> Gain14/1  "Om"
  Gain14/1 -> Trigonometric Function6/1
  Constant26/1 -> Product16/1
  Trigonometric Function6/1 -> Product16/2
  Add8/1 -> Gain15/1  "L"
  Gain15/1 -> Trigonometric Function7/1
  Trigonometric Function7/1 -> Product17/2
  Constant28/1 -> Product17/1
  Product16/1 -> Add9/1
  Product17/1 -> Add9/2
  Subtract1/1 -> Gain16/1  "eps"
  Gain16/1 -> Trigonometric Function8/1
  Add9/1 -> Product18/1  "delta_psi"
  Trigonometric Function8/1 -> Product18/2
  Product18/1 -> Add7/2  "eqeq"
  Math Function/1 -> Add7/1  "GMST"
  Add7/1 -> Gain17/1
  Matrix Concatenate1/1 -> Switch/3
  Constant27/1 -> Matrix Concatenate1/3
  Gain17/1 -> Trigonometric Function10/1, Trigonometric Function9/1  "GAST"
  Trigonometric Function10/2 -> Vector Concatenate3/1
  Trigonometric Function10/1 -> Gain24/1
  Constant29/1 -> Vector Concatenate3/3
  Trigonometric Function9/1 -> Vector Concatenate4/1
  Trigonometric Function9/2 -> Vector Concatenate4/2
  Constant30/1 -> Vector Concatenate4/3
  Vector Concatenate4/1 -> Matrix Concatenate1/2
  Vector Concatenate3/1 -> Matrix Concatenate1/1
  Constant32/1 -> Product19/2
  Product19/1 -> Product10/1, Product9/2, Product10/2
  [d_no_hours] -> Product13/2
  [d_no_hours] -> Product12/2
  [t] -> Product20/1
  Constant33/1 -> Product20/2
  [ut_hours] -> Gain20/1
  Product20/1 -> Sum8/1
  Gain20/1 -> Sum8/2
  Sum8/1 -> [d_no_hours]
  [ut_hours] -> Gain23/1
  Sum7/1 -> Product19/1
  Gain19/1 -> Sum7/1
  Gain23/1 -> Sum7/2
  Gain24/1 -> Vector Concatenate3/2
  [d] -> Gain18/1
  Gain18/1 -> [sec_xjdate]
  Constant31/1 -> Math Function3/2
  Math Function3/1 -> Divide/1
  Constant34/1 -> Divide/2
  Constant35/1 -> Subtract3/2
  Subtract3/1 -> Math Function3/1
  [sec_xjdate] -> Gain19/1
  [sec_xjdate] -> Subtract3/1

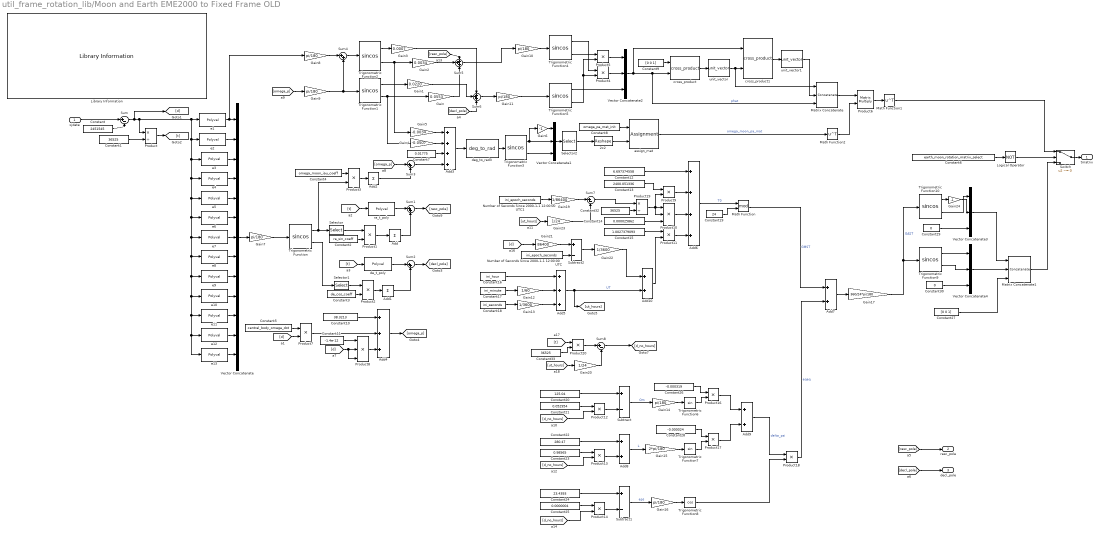
== system util_frame_rotation_lib/Moon and Earth EME2000 to Fixed Frame OLD ==
  xjdate : Inport
  2x2 : Reshape  OutputDimensionality=Customize  OutputDimensions=[2,2]
  Add : Sum  Inputs=+
  Add1 : Sum  Inputs=+
  Add{7..10} (4 alike) : Sum  Inputs=2
  Add2 : Sum  Inputs=+
  Add3 : Sum  Inputs=4
  Add4 : Sum  Inputs=3
  Add5 : Sum  Inputs=3
  Add6 : Sum  Inputs=4
  Constant : Constant  Value=2451545
  Constant1 : Constant  Value=36525
  Constant10 : Constant  Value=38.3213
  Constant11 : Constant  Value=-1.4e-12
  Constant12 : Constant  Value=6.697374558
  Constant13 : Constant  Value=2400.051336
  Constant14 : Constant  Value=0.000025862
  Constant15 : Constant  Value=1.0027379093
  Constant16 : Constant  Value=ini_hour
  Constant17 : Constant  Value=ini_minute
  Constant18 : Constant  Value=ini_seconds
  Constant19 : Constant  Value=24
  Constant2 : Constant  Value=ra_sin_coeff
  Constant20 : Constant  Value=125.04
  Constant21 : Constant  Value=0.052954
  Constant22 : Constant  Value=280.47
  Constant23 : Constant  Value=0.98565
  Constant24 : Constant  Value=23.4393
  Constant25 : Constant  Value=0.0000004
  Constant26 : Constant  Value=-0.000319
  Constant27 : Constant  Value=[0 0 1]
  Constant28 : Constant  Value=-0.000024
  Constant29 : Constant  Value=0
  Constant3 : Constant  Value=de_cos_coeff
  Constant30 : Constant  Value=0
  Constant32 : Constant  Value=36525
  Constant33 : Constant  Value=36525
  Constant4 : Constant  Value=omega_moon_iau_coeff
  Constant5 : Constant  Value=central_body_omega_dot
  Constant6 : Constant  Value=earth_moon_rotation_matrix_select
  Constant7 : Constant  Value=0.01775
  Constant8 : Constant  Value=omega_pa_mat_init
  Constant9 : Constant  Value=[0 0 1]
  Gain : Gain  Gain=0.0553
  Gain1 : Gain  Gain=0.0220
  Gain{7..11,14,16} (7 alike) : Gain  Gain=pi/180
  Gain12 : Gain  Gain=1/60
  Gain13 : Gain  Gain=1/3600
  Gain15 : Gain  Gain=2*pi/180
  Gain17 : Gain  Gain=360/24*pi/180
  Gain19 : Gain  Gain=1/86400
  Gain2 : Gain  Gain=0.0034
  Gain20 : Gain  Gain=1/24
  Gain21 : Gain  Gain=86400
  Gain22 : Gain  Gain=1/3600
  Gain23 : Gain  Gain=1/24
  Gain24 : Gain  Gain=-1
  Gain3 : Gain  Gain=0.0007
  Gain4 : Gain  Gain=-0.0507
  Gain5 : Gain  Gain=-0.0034
  Gain6 : Gain  Gain=-1
  Library Information : util_info_lib/Library Information  owner='escrane'
  Logical Operator : Logic  Operator=NOT  AllPortsSameDT=off  OutDataTypeStr=boolean
  Math Function : Math  Operator=mod  SaturateOnIntegerOverflow=on
  Math Function1 : Math  Operator=transpose  SaturateOnIntegerOverflow=on
  Math Function2 : Math  Operator=transpose  SaturateOnIntegerOverflow=on
  Matrix Concatenate : Concatenate  NumInputs=3  Mode=Multidimensional array  ConcatenateDimension=2
  Matrix Concatenate1 : Concatenate  NumInputs=3  Mode=Multidimensional array  ConcatenateDimension=2
  Number of Seconds Since 2000-1-1 12:00:00 UTC : Constant  Description=|  Value=ini_epoch_seconds
      | Number of Seconds                   
      | July 4, 2014 22:40:00 UTC           
      | Calculate on Web Site:              
      | www.mbari.org/staff/rich/utccalc.htm
  Number of Seconds Since 2000-1-1 12:00:00 UTC1 : Constant  Description=|  Value=ini_epoch_seconds
      | Number of Seconds                   
      | July 4, 2014 22:40:00 UTC           
      | Calculate on Web Site:              
      | www.mbari.org/staff/rich/utccalc.htm
  Product : Product  Inputs=*/
  Product{1..5,7,9,11..14,16..18,20} (15 alike) : Product
  Product10 : Product  Inputs=3
  Product19 : Product  Inputs=*/
  Product6 : Product  Multiplication=Matrix(*)
  Product8 : Product  Inputs=3
  Selector : Selector  InputPortWidth=13  IndexOptions=Index vector (dialog)  Indices=[1 2 3 4 6 10 13]  OutputSizes=1
  Selector1 : Selector  InputPortWidth=13  IndexOptions=Index vector (dialog)  Indices=[1 2 3 4 6 7 10 13]  OutputSizes=1
  Selector2 : Selector  InputPortWidth=3  IndexOptions=Index vector (dialog)  Indices=[3 1 2 3]  OutputSizes=1
  Subtract : Sum  Inputs=+-
  Subtract1 : Sum  Inputs=+-
  Subtract2 : Sum  Inputs=+-
  Sum : Sum  Inputs=|+-
  Sum{1..4} (4 alike) : Sum  Inputs=|++
  Sum5 : Sum  Inputs=+++
  Sum6 : Sum  Inputs=+++
  Sum7 : Sum  Inputs=|+-
  Sum8 : Sum  Inputs=|+-
  Switch : Switch  Criteria=u2 ~= 0
  Trigonometric Function{,1..5,9..10} (8 alike) : Trigonometry  Operator=sincos
  Trigonometric Function6 : Trigonometry
  Trigonometric Function7 : Trigonometry
  Trigonometric Function8 : Trigonometry  Operator=cos
  Vector Concatenate : Concatenate  NumInputs=13
  Vector Concatenate{1..4} (4 alike) : Concatenate  NumInputs=3
  assign_mat : Assignment  NumberOfDimensions=2  IndexOptions=Index vector (dialog),Index vector (dialog)  Indices=[1 2],[1 2]  OutputSizes=1,1
  cross_product : util_common_lib/cross_product  SystemSampleTime=-1
  cross_product1 : util_common_lib/cross_product  SystemSampleTime=-1
  de_t_poly : Polyval  Coefs=de_t_poly
  deg_to_rad3 : util_common_lib/deg_to_rad  SystemSampleTime=-1
  e1 : Polyval  Coefs=e1coeff
  e10 : Polyval  Coefs=e10coeff
  e11 : Polyval  Coefs=e11coeff
  e12 : Polyval  Coefs=e12coeff
  e13 : Polyval  Coefs=e13coeff
  e2 : Polyval  Coefs=e2coeff
  e3 : Polyval  Coefs=e3coeff
  e4 : Polyval  Coefs=e4coeff
  e5 : Polyval  Coefs=e5coeff
  e6 : Polyval  Coefs=e6coeff
  e7 : Polyval  Coefs=e7coeff
  e8 : Polyval  Coefs=e8coeff
  e9 : Polyval  Coefs=e9coeff
  ra_t_poly : Polyval  Coefs=ra_t_poly
  unit_vector : util_common_lib/unit_vector  SystemSampleTime=-1
  unit_vector1 : util_common_lib/unit_vector  SystemSampleTime=-1
  tmatrix : Outport
  rasc_pole : Outport  Port=2
  decl_pole : Outport  Port=3
  wires:
  [decl_pole] -> decl_pole/1
  [rasc_pole] -> rasc_pole/1
  Math Function2/1 -> Product6/2
  Trigonometric Function5/2 -> Product5/2, Product4/2
  Gain3/1 -> Sum6/1
  Gain1/1 -> Sum6/2
  Gain2/1 -> Sum5/2
  Gain/1 -> Sum5/3
  Product6/1 -> Math Function1/1
  Matrix Concatenate/1 -> Product6/1
  unit_vector1/1 -> Matrix Concatenate/2
  cross_product1/1 -> unit_vector1/1
  unit_vector/1 -> cross_product1/2, Matrix Concatenate/1
  cross_product/1 -> unit_vector/1
  Constant9/1 -> cross_product/1
  Vector Concatenate2/1 -> cross_product/2, Matrix Concatenate/3, cross_product1/1  "phat"
  Product4/1 -> Vector Concatenate2/2
  Product5/1 -> Vector Concatenate2/1
  Trigonometric Function4/2 -> Product5/1
  Trigonometric Function5/1 -> Vector Concatenate2/3
  Trigonometric Function4/1 -> Product4/1
  Gain11/1 -> Trigonometric Function5/1
  Gain10/1 -> Trigonometric Function4/1
  assign_mat/1 -> Math Function2/1  "omega_moon_pa_mat"
  Constant8/1 -> assign_mat/1
  2x2/1 -> assign_mat/2
  Selector2/1 -> 2x2/1
  Vector Concatenate1/1 -> Selector2/1
  Gain6/1 -> Vector Concatenate1/1
  Trigonometric Function3/1 -> Vector Concatenate1/2, Gain6/1
  Trigonometric Function3/2 -> Vector Concatenate1/3
  deg_to_rad3/1 -> Trigonometric Function3/1
  Add3/1 -> deg_to_rad3/1
  Constant7/1 -> Add3/3
  Gain4/1 -> Add3/2
  Gain5/1 -> Add3/1
  Sum6/1 -> Gain11/1
  Sum5/1 -> Gain10/1
  [rasc_pole] -> Sum5/1
  [decl_pole] -> Sum6/3
  Trigonometric Function2/2 -> Gain5/1, Gain2/1
  Trigonometric Function2/1 -> Gain3/1
  Trigonometric Function1/1 -> Gain1/1
  Trigonometric Function1/2 -> Gain/1, Gain4/1
  Sum4/1 -> Trigonometric Function2/1
  Gain8/1 -> Sum4/1
  Gain9/1 -> Trigonometric Function1/1, Sum4/2
  [omega_p] -> Gain9/1
  Sum3/1 -> Add3/4
  Add2/1 -> Sum3/2
  Product3/1 -> Add2/1
  Constant4/1 -> Product3/1
  Sum2/1 -> [decl_pole]
  Add1/1 -> Sum2/2
  de_t_poly/1 -> Sum2/1
  Product2/1 -> Add1/1
  Constant3/1 -> Product2/2
  Selector1/1 -> Product2/1
  [t] -> de_t_poly/1
  Sum1/1 -> [rasc_pole]
  Add/1 -> Sum1/2
  ra_t_poly/1 -> Sum1/1
  Product1/1 -> Add/1
  Constant2/1 -> Product1/2
  Selector/1 -> Product1/1
  [t] -> ra_t_poly/1
  Trigonometric Function/2 -> Selector1/1
  Trigonometric Function/1 -> Selector/1, Product3/2
  Gain7/1 -> Trigonometric Function/1
  Vector Concatenate/1 -> Gain7/1
  e13/1 -> Vector Concatenate/13
  e12/1 -> Vector Concatenate/12
  e11/1 -> Vector Concatenate/11
  e10/1 -> Vector Concatenate/10
  e9/1 -> Vector Concatenate/9
  e8/1 -> Vector Concatenate/8
  e7/1 -> Vector Concatenate/7
  e6/1 -> Vector Concatenate/6
  e5/1 -> Vector Concatenate/5
  e4/1 -> Vector Concatenate/4
  e3/1 -> Vector Concatenate/3
  e2/1 -> Vector Concatenate/2
  e1/1 -> Vector Concatenate/1, Gain8/1
  Sum/1 -> [d], Product/1, e1/1, e2/1, e3/1, e4/1, e5/1, e6/1, e7/1, e8/1, e9/1, e11/1, e12/1, e13/1, e10/1
  Product/1 -> [t]
  Constant1/1 -> Product/2
  Constant/1 -> Sum/2
  xjdate/1 -> Sum/1
  Constant5/1 -> Product7/1
  [d] -> Product7/2
  Constant11/1 -> Product8/1
  [d] -> Product8/3, Product8/2
  Constant10/1 -> Add4/1
  Product7/1 -> Add4/2
  Product8/1 -> Add4/3
  Add4/1 -> [omega_p]
  [omega_p] -> Sum3/1
  Constant6/1 -> Logical Operator/1
  Logical Operator/1 -> Switch/2
  Switch/1 -> tmatrix/1
  Math Function1/1 -> Switch/1
  Constant16/1 -> Add5/1
  Constant18/1 -> Gain13/1
  Constant17/1 -> Gain12/1
  Gain12/1 -> Add5/2
  Gain13/1 -> Add5/3
  Constant12/1 -> Add6/1
  Constant13/1 -> Product9/1
  Product9/1 -> Add6/2
  Constant14/1 -> Product10/3
  Product10/1 -> Add6/3
  Constant15/1 -> Product11/1
  Add5/1 -> Add10/2, [ut_hours]  "UT"
  Product11/1 -> Add6/4
  Constant19/1 -> Math Function/2
  Add6/1 -> Math Function/1  "T0"
  Constant20/1 -> Subtract/1
  Product12/1 -> Subtract/2
  Constant21/1 -> Product12/1
  Constant22/1 -> Add8/1
  Product13/1 -> Add8/2
  Constant23/1 -> Product13/1
  Constant24/1 -> Subtract1/1
  Product14/1 -> Subtract1/2
  Constant25/1 -> Product14/1
  [d_no_hours] -> Product14/2
  Subtract/1 -> Gain14/1  "Om"
  Gain14/1 -> Trigonometric Function6/1
  Constant26/1 -> Product16/1
  Trigonometric Function6/1 -> Product16/2
  Add8/1 -> Gain15/1  "L"
  Gain15/1 -> Trigonometric Function7/1
  Trigonometric Function7/1 -> Product17/2
  Constant28/1 -> Product17/1
  Product16/1 -> Add9/1
  Product17/1 -> Add9/2
  Subtract1/1 -> Gain16/1  "eps"
  Gain16/1 -> Trigonometric Function8/1
  Add9/1 -> Product18/1  "delta_psi"
  Trigonometric Function8/1 -> Product18/2
  Product18/1 -> Add7/2  "eqeq"
  Math Function/1 -> Add7/1  "GMST"
  Add7/1 -> Gain17/1
  Matrix Concatenate1/1 -> Switch/3
  Constant27/1 -> Matrix Concatenate1/3
  Gain17/1 -> Trigonometric Function10/1, Trigonometric Function9/1  "GAST"
  Trigonometric Function10/2 -> Vector Concatenate3/1
  Trigonometric Function10/1 -> Gain24/1
  Constant29/1 -> Vector Concatenate3/3
  Trigonometric Function9/1 -> Vector Concatenate4/1
  Trigonometric Function9/2 -> Vector Concatenate4/2
  Constant30/1 -> Vector Concatenate4/3
  Vector Concatenate4/1 -> Matrix Concatenate1/2
  Vector Concatenate3/1 -> Matrix Concatenate1/1
  Constant32/1 -> Product19/2
  Product19/1 -> Product10/1, Product9/2, Product10/2
  [d_no_hours] -> Product13/2
  [d_no_hours] -> Product12/2
  Add10/1 -> Product11/2
  Gain22/1 -> Add10/1
  [d] -> Gain21/1
  Number of Seconds Since 2000-1-1 12:00:00 UTC/1 -> Subtract2/2
  Gain21/1 -> Subtract2/1
  Subtract2/1 -> Gain22/1
  [t] -> Product20/1
  Constant33/1 -> Product20/2
  [ut_hours] -> Gain20/1
  Product20/1 -> Sum8/1
  Gain20/1 -> Sum8/2
  Sum8/1 -> [d_no_hours]
  Number of Seconds Since 2000-1-1 12:00:00 UTC1/1 -> Gain19/1
  [ut_hours] -> Gain23/1
  Sum7/1 -> Product19/1
  Gain19/1 -> Sum7/1
  Gain23/1 -> Sum7/2
  Gain24/1 -> Vector Concatenate3/2

== system util_frame_rotation_lib/Topocentric to J2000 Vector Transformation  ==
  Clock Update : Inport
  Vector  Topocentric : Inport  Port=2
  Constant10 : Constant  Value=ini_tgt_landing_mcmf_pos
  Library Information : util_info_lib/Library Information  owner='NONE'
  MCMF to J2000 Transformation Quaternion : util_frame_rotation_lib/MCMF to J2000  Transformation Quaternion
  Moon Rotation Rate in MCMF : Constant  Value=ini_quat_mcmf_to_topo
  Subtract1 : Sum
  quaternion_conjugate q_topo_to_mcmf : util_quat_lib/quaternion_conjugate  SystemSampleTime=-1
  quaternion_frame_transformation v_mcmf : util_quat_lib/quaternion_frame_transformation  SystemSampleTime=-1
  qjMCMF to J2000 : Outport
  Vector J2000 : Outport  Port=2
  wires:
  Vector  Topocentric/1 -> quaternion_frame_transformation v_mcmf/1
  Moon Rotation Rate in MCMF/1 -> quaternion_conjugate q_topo_to_mcmf/1
  quaternion_conjugate q_topo_to_mcmf/1 -> quaternion_frame_transformation v_mcmf/2
  MCMF to J2000 Transformation Quaternion/2 -> Vector J2000/1
  MCMF to J2000 Transformation Quaternion/1 -> qjMCMF to J2000/1
  Clock Update/1 -> MCMF to J2000 Transformation Quaternion/1
  Constant10/1 -> Subtract1/1
  quaternion_frame_transformation v_mcmf/1 -> Subtract1/2
  Subtract1/1 -> MCMF to J2000 Transformation Quaternion/2

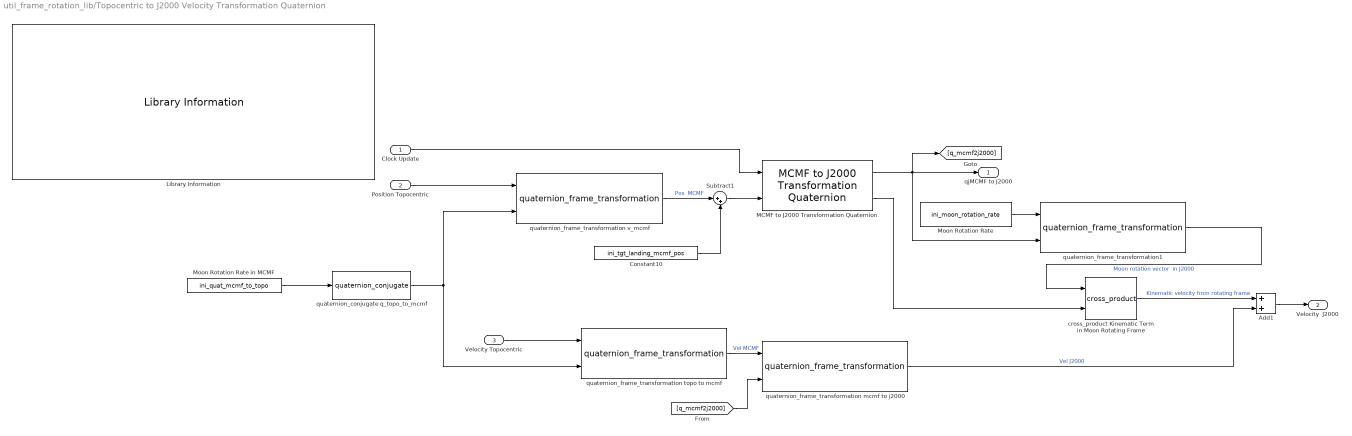
== system util_frame_rotation_lib/Topocentric to J2000 Velocity Transformation Quaternion ==
  Clock Update : Inport
  Position Topocentric : Inport  Port=2
  Velocity Topocentric : Inport  Port=3
  Add1 : Sum
  Constant10 : Constant  Value=ini_tgt_landing_mcmf_pos
  Library Information : util_info_lib/Library Information  owner='NONE'
  MCMF to J2000 Transformation Quaternion : util_frame_rotation_lib/MCMF to J2000  Transformation Quaternion
  Moon Rotation Rate : Constant  Value=ini_moon_rotation_rate
  Moon Rotation Rate in MCMF : Constant  Value=ini_quat_mcmf_to_topo
  Subtract1 : Sum  Inputs=|++
  cross_product Kinematic Term in Moon Rotating Frame : util_common_lib/cross_product  SystemSampleTime=-1
  quaternion_conjugate q_topo_to_mcmf : util_quat_lib/quaternion_conjugate  SystemSampleTime=-1
  quaternion_frame_transformation mcmf to j2000 : util_quat_lib/quaternion_frame_transformation  SystemSampleTime=-1
  quaternion_frame_transformation topo to mcmf : util_quat_lib/quaternion_frame_transformation  SystemSampleTime=-1
  quaternion_frame_transformation v_mcmf : util_quat_lib/quaternion_frame_transformation  SystemSampleTime=-1
  quaternion_frame_transformation1 : util_quat_lib/quaternion_frame_transformation  SystemSampleTime=-1
  qjMCMF to J2000 : Outport
  Velocity  J2000 : Outport  Port=2
  wires:
  Position Topocentric/1 -> quaternion_frame_transformation v_mcmf/1
  Moon Rotation Rate in MCMF/1 -> quaternion_conjugate q_topo_to_mcmf/1
  quaternion_conjugate q_topo_to_mcmf/1 -> quaternion_frame_transformation v_mcmf/2, quaternion_frame_transformation topo to mcmf/2
  MCMF to J2000 Transformation Quaternion/1 -> [q_mcmf2j2000], quaternion_frame_transformation1/2, qjMCMF to J2000/1
  quaternion_frame_transformation v_mcmf/1 -> Subtract1/1  "Pos  MCMF"
  Clock Update/1 -> MCMF to J2000 Transformation Quaternion/1
  Velocity Topocentric/1 -> quaternion_frame_transformation topo to mcmf/1
  quaternion_frame_transformation topo to mcmf/1 -> quaternion_frame_transformation mcmf to j2000/1  "Vel MCMF"
  Moon Rotation Rate/1 -> quaternion_frame_transformation1/1
  quaternion_frame_transformation1/1 -> cross_product Kinematic Term in Moon Rotating Frame/1  "Moon rotation vector  in J2000"
  MCMF to J2000 Transformation Quaternion/2 -> cross_product Kinematic Term in Moon Rotating Frame/2
  Add1/1 -> Velocity  J2000/1
  quaternion_frame_transformation mcmf to j2000/1 -> Add1/2  "Vel J2000"
  cross_product Kinematic Term in Moon Rotating Frame/1 -> Add1/1  "Kinematic velocity from rotating frame"
  [q_mcmf2j2000] -> quaternion_frame_transformation mcmf to j2000/2
  Subtract1/1 -> MCMF to J2000 Transformation Quaternion/2
  Constant10/1 -> Subtract1/2

== system util_frame_rotation_lib/Topocentric to MCMF ==
  Vector  Topocentric : Inport
  Library Information : util_info_lib/Library Information  owner='NONE'
  Moon Rotation Rate in MCMF : Constant  Value=ini_quat_mcmf_to_topo
  quaternion_conjugate q_topo_to_mcmf : util_quat_lib/quaternion_conjugate  SystemSampleTime=-1
  quaternion_frame_transformation v_mcmf : util_quat_lib/quaternion_frame_transformation  SystemSampleTime=-1
  Vector MCMF : Outport
  q_topo2mcmf : Outport  Port=2
  wires:
  Vector  Topocentric/1 -> quaternion_frame_transformation v_mcmf/1
  Moon Rotation Rate in MCMF/1 -> quaternion_conjugate q_topo_to_mcmf/1
  quaternion_conjugate q_topo_to_mcmf/1 -> q_topo2mcmf/1, quaternion_frame_transformation v_mcmf/2
  quaternion_frame_transformation v_mcmf/1 -> Vector MCMF/1  "Vector MCMF"

== system util_frame_rotation_lib/Topocentric to MCMF Position ==
  Pos  Topocentric : Inport
  Constant10 : Constant  Value=ini_tgt_landing_mcmf_pos
  Library Information : util_info_lib/Library Information  owner='NONE'
  Moon Rotation Rate in MCMF : Constant  Value=ini_quat_mcmf_to_topo
  Subtract1 : Sum
  quaternion_conjugate q_topo_to_mcmf : util_quat_lib/quaternion_conjugate  SystemSampleTime=-1
  quaternion_frame_transformation v_mcmf : util_quat_lib/quaternion_frame_transformation  SystemSampleTime=-1
  Vector MCMF : Outport
  q_topo2mcmf : Outport  Port=2
  wires:
  Pos  Topocentric/1 -> quaternion_frame_transformation v_mcmf/1
  Moon Rotation Rate in MCMF/1 -> quaternion_conjugate q_topo_to_mcmf/1
  quaternion_conjugate q_topo_to_mcmf/1 -> q_topo2mcmf/1, quaternion_frame_transformation v_mcmf/2
  Constant10/1 -> Subtract1/1
  quaternion_frame_transformation v_mcmf/1 -> Subtract1/2  "Vector MCMF"
  Subtract1/1 -> Vector MCMF/1

== system util_frame_rotation_lib/calc_cos_elevation ==
  quat : Inport
  Demux2 : Demux  Outputs=[2 1 1]
  Gain : Gain  Gain=2
  Library Information : util_info_lib/Library Information  owner='NONE'
  Sum : Sum  Inputs=|++
  Sum1 : Sum  Inputs=|+-
  Terminator : Terminator
  inertial_z_axis1 : Constant
  range_true1 : Product  RndMeth=Zero
  range_true2 : Product  RndMeth=Zero
  cos_el : Outport
  wires:
  Demux2/2 -> range_true1/1, range_true1/2
  Demux2/3 -> range_true2/1, range_true2/2
  range_true1/1 -> Sum/1
  range_true2/1 -> Sum/2
  Sum/1 -> Gain/1
  inertial_z_axis1/1 -> Sum1/2
  Gain/1 -> Sum1/1
  Sum1/1 -> cos_el/1
  quat/1 -> Demux2/1
  Demux2/1 -> Terminator/1
